simulink model "Cv_8_simulink"  (R2024a)
settings: Solver=FixedStepAuto  StartTime=0.0  StopTime=10.0  FixedStep=1e-3  RelTol=1e-3
values from neighbouring files (symbols this model uses):
  A2 = [0   , 1 ... (first row only)    [Cv_8.m]
  B2 = [0; 1/m]    [Cv_8.m]
  C2 = eye(2,2)    [Cv_8.m]
  D2 = zeros(2,1)    [Cv_8.m]
  den = [m, b, k]    [Cv_8.m]
  F0 = 1    [Cv_8.m]
  num = [1]    [Cv_8.m]
  omega = 5    [Cv_8.m]
  v0 = 0    [Cv_8.m]
  x0 = 0    [Cv_8.m]
undefined symbols (not defined in the file or in its folder): A1, B1, C1, D1
settings Model: Creator=221208  LastModifiedBy=Miloš Uhlíř
settings ModelReferenceCC: EnableRefExpFcnMdlSchedulingChecks=on
settings RTWCC: GPUComputeCapability=3.5

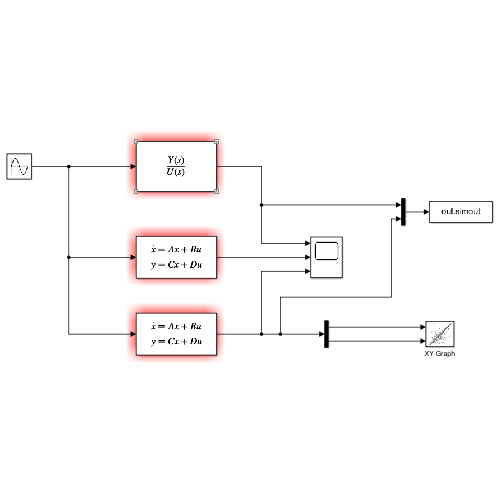
[thumbnail: Simulink's stored preview of the top-level diagram]
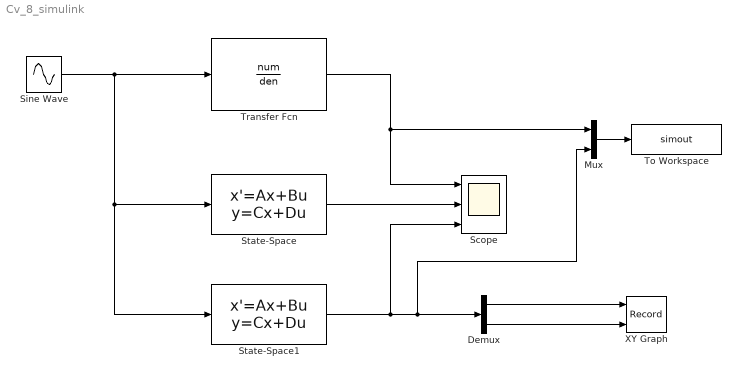
== system Cv_8_simulink ==
  Demux : Demux  Outputs=2
  Mux : Mux  Inputs=2
  Scope : Scope  NumInputPorts=3
  Sine Wave : Sin  Amplitude=F0  Frequency=omega  SampleTime=0
  State-Space : StateSpace  A=A1  B=B1  C=C1  D=D1  InitialCondition=[v0 x0]
  State-Space1 : StateSpace  A=A2  B=B2  C=C2  D=D2  InitialCondition=[x0 v0]
  To Workspace : ToWorkspace  VariableName=simout  SaveFormat=Timeseries  SampleTime=-1
  Transfer Fcn : TransferFcn  Numerator=num  Denominator=den
  XY Graph : Record  FileSettingsInternal="{\"entries\":[{\"content\":{\"excelSettings\":{\"content\":{},\"type\":\"Streamout.ExcelSettings\"}},\"type\":\"Streamout.FileSettingStorage\",\"uuid\":\"\"}],\"packageUris\":[\"http:\\/\\/schema.mathworks.com\\/mf0\\/streamout_blocks\\/R2020a\"],\"version\":\"1.0\"}"  Layout=[1 1]  SignalsInternal="{\"entries\":[{\"content\":{\"signals\":[{\"content\":{\"blockPath\":[],\"dimensions\":[1],\"domain\":\"\",\"lineColor\":\"#a2142f\",\"plots\":[ 1 ],\"port\":1,\"signalID\":1,\"signalName\":\"Demux:1\"},\"type\":\"RecordBlkView.Signal\",\"uuid\":\"\"},{\"content\":{\"blockPath\":[],\"dimensions\":[1],\"domain\":\"\",\"lineColor\":\"#139fff\",\"plots\":[ 1 ],\"port\":2,\"signalID\":2,\"signalName\":\"Demux:2\"},\"type\":\"RecordBlkView.Signal\",\"uuid\":\"\"}]},\"type\":\"RecordBlkView.InputSignals\",\"uuid\":\"\"}],\"packageUris\":[\"http:\\/\\/schema.mathworks.com\\/mf0\\/streamout_blocks\\/R2020a\"],\"version\":\"1.0\"}"  VisualizationBindings="{\"xyplotplugin\":{\"info\":[{\"series\":[{\"bindingParametersList\":[{\"parameter\":\"X-Axis\",\"signalID\":1,\"signalName\":\"Demux:1\"},{\"parameter\":\"Y-Axis\",\"signalID\":2,\"signalName\":\"Demux:2\"}],\"seriesID\":0}],\"subplotID\":1}]}}"  CompatibilityTag=XY
  wires:
  Sine Wave/1 -> State-Space1/1, State-Space/1, Transfer Fcn/1
  Transfer Fcn/1 -> Mux/1, Scope/1
  State-Space/1 -> Scope/2
  State-Space1/1 -> Mux/2, Demux/1, Scope/3
  Demux/1 -> XY Graph/1
  Demux/2 -> XY Graph/2
  Mux/1 -> To Workspace/1
